simulink model "MCU_SpeedCal"  (R2022b)
settings: Solver=FixedStepDiscrete  StartTime=0.0  StopTime=10.0  RelTol=1e-3
undefined symbols (not defined in the file or in its folder): ParamCfg_RotateNp_u16, ParamCfg_ZeroTorqueNoworkSpeed_u16, ParamCfg_ZeroTorqueWorkSpeed_u16, POWER_ON
libraries: simulink x3
settings Model: DataDictionary=MCU_SpeedCal_Sldd.sldd  Creator=ZYH  LastModifiedBy=ZYH
settings OptimizationCC: DefaultParameterBehavior=Inlined  EnhancedBackFolding=on  PassReuseOutputArgsAs=Individual arguments  ZeroExternalMemoryAtStartup=off  ZeroInternalMemoryAtStartup=off  OptimizeBlockOrder=speed  DifferentSizesBufferReuse=on  OptimizationCustomize=off  EfficientTunableParamExpr=on
settings DebuggingCC: ParameterTunabilityLossMsg=error
settings SFSimCC: MATLABDynamicMemAlloc=off
settings RTWCC: Description=Embedded Coder  SystemTargetFile=ert.tlc  GenCodeOnly=on  TemplateMakefile=ert_default_tmf
settings CodeAppCC: ForceParamTrailComments=on  IgnoreCustomStorageClasses=off  OperatorAnnotations=on  SimulinkDataObjDesc=on  SFDataObjDesc=on  InsertBlockDesc=on
settings ERTTargetCC: TargetLangStandard=C99 (ISO)  GenerateSampleERTMain=on  InlinedParameterPlacement=NonHierarchical  ERTCustomFileTemplate=example_file_process.tlc

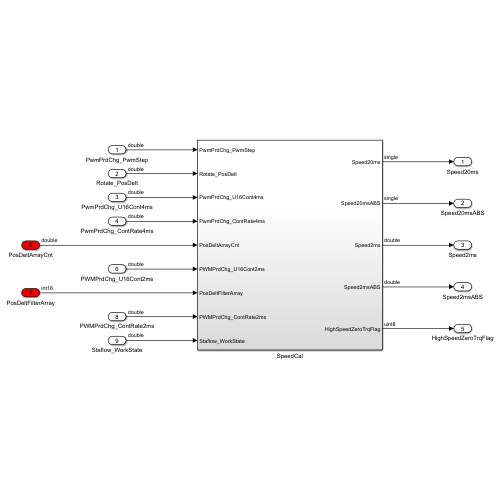
[thumbnail: Simulink's stored preview of the top-level diagram]
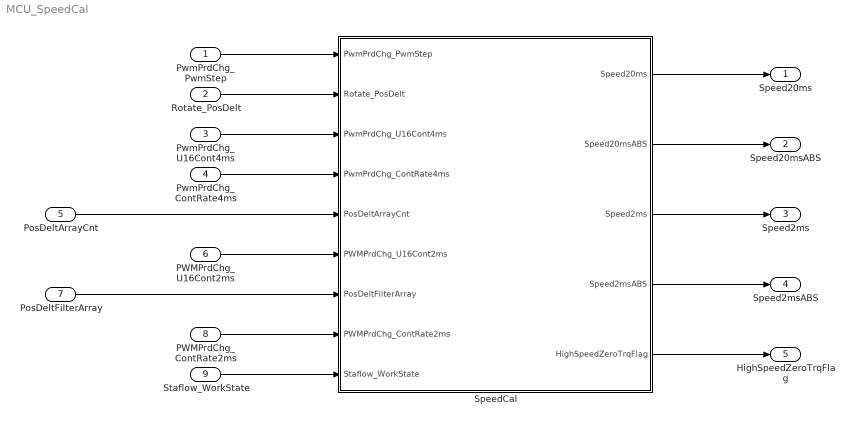
== system MCU_SpeedCal ==
  PwmPrdChg_PwmStep : Inport
  Rotate_PosDelt : Inport  Port=2
  PwmPrdChg_U16Cont4ms : Inport  Port=3
  PwmPrdChg_ContRate4ms : Inport  Port=4
  PosDeltArrayCnt : Inport  Port=5
  PWMPrdChg_U16Cont2ms : Inport  Port=6
  PosDeltFilterArray : Inport  Port=7
  PWMPrdChg_ContRate2ms : Inport  Port=8
  Staflow_WorkState : Inport  Port=9
  SpeedCal : Subsystem
  Speed20ms : Outport
  Speed20msABS : Outport  Port=2
  Speed2ms : Outport  Port=3
  Speed2msABS : Outport  Port=4
  HighSpeedZeroTrqFlag : Outport  Port=5
  wires:
  PwmPrdChg_PwmStep/1 -> SpeedCal/1(PwmPrdChg_PwmStep)
  Rotate_PosDelt/1 -> SpeedCal/2(Rotate_PosDelt)
  PwmPrdChg_U16Cont4ms/1 -> SpeedCal/3(PwmPrdChg_U16Cont4ms)
  PwmPrdChg_ContRate4ms/1 -> SpeedCal/4(PwmPrdChg_ContRate4ms)
  PosDeltArrayCnt/1 -> SpeedCal/5(PosDeltArrayCnt)
  PWMPrdChg_U16Cont2ms/1 -> SpeedCal/6(PWMPrdChg_U16Cont2ms)
  PosDeltFilterArray/1 -> SpeedCal/7(PosDeltFilterArray)
  PWMPrdChg_ContRate2ms/1 -> SpeedCal/8(PWMPrdChg_ContRate2ms)
  SpeedCal/1(Speed20ms) -> Speed20ms/1
  SpeedCal/2(Speed20msABS) -> Speed20msABS/1
  SpeedCal/3(Speed2ms) -> Speed2ms/1
  SpeedCal/4(Speed2msABS) -> Speed2msABS/1
  SpeedCal/5(HighSpeedZeroTrqFlag) -> HighSpeedZeroTrqFlag/1
  Staflow_WorkState/1 -> SpeedCal/9(Staflow_WorkState)

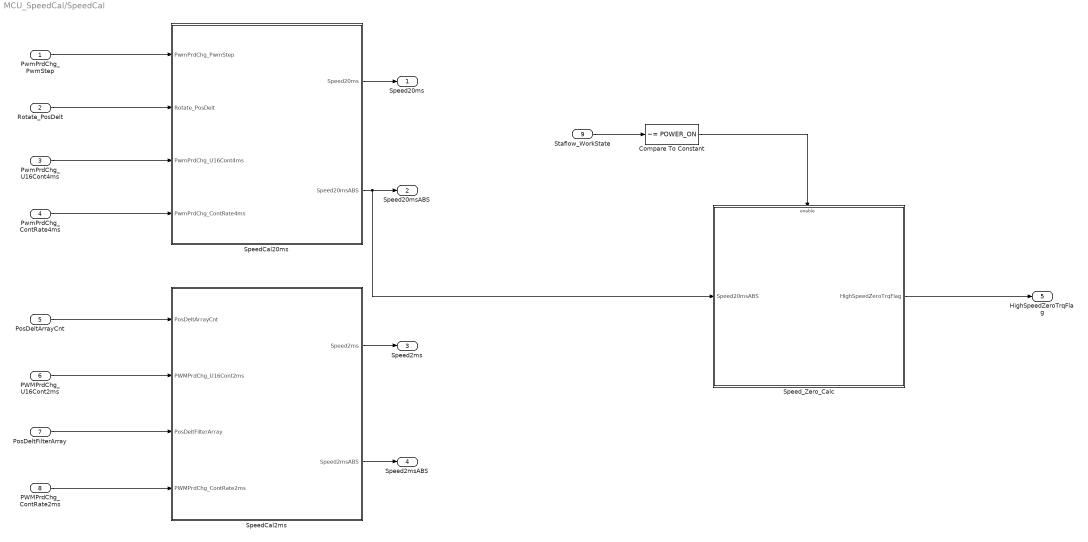
== system MCU_SpeedCal/SpeedCal ==
  PwmPrdChg_PwmStep : Inport
  Rotate_PosDelt : Inport  Port=2
  PwmPrdChg_U16Cont4ms : Inport  Port=3
  PwmPrdChg_ContRate4ms : Inport  Port=4
  PosDeltArrayCnt : Inport  Port=5
  PWMPrdChg_U16Cont2ms : Inport  Port=6
  PosDeltFilterArray : Inport  Port=7
  PWMPrdChg_ContRate2ms : Inport  Port=8
  Staflow_WorkState : Inport  Port=9
  Compare To Constant : simulink/Logic and Bit Operations/Compare To Constant  relop=~=  const=POWER_ON  OutDataTypeStr=boolean
  SpeedCal20ms : Subsystem
  SpeedCal2ms : Subsystem
  Speed_Zero_Calc : Subsystem
  Speed20ms : Outport
  Speed20msABS : Outport  Port=2
  Speed2ms : Outport  Port=3
  Speed2msABS : Outport  Port=4
  HighSpeedZeroTrqFlag : Outport  Port=5
  wires:
  PwmPrdChg_PwmStep/1 -> SpeedCal20ms/1(PwmPrdChg_PwmStep)
  Rotate_PosDelt/1 -> SpeedCal20ms/2(Rotate_PosDelt)
  PwmPrdChg_U16Cont4ms/1 -> SpeedCal20ms/3(PwmPrdChg_U16Cont4ms)
  PwmPrdChg_ContRate4ms/1 -> SpeedCal20ms/4(PwmPrdChg_ContRate4ms)
  SpeedCal20ms/1(Speed20ms) -> Speed20ms/1
  SpeedCal20ms/2(Speed20msABS) -> Speed20msABS/1, Speed_Zero_Calc/1(Speed20msABS)
  PosDeltArrayCnt/1 -> SpeedCal2ms/1(PosDeltArrayCnt)
  PWMPrdChg_U16Cont2ms/1 -> SpeedCal2ms/2(PWMPrdChg_U16Cont2ms)
  PosDeltFilterArray/1 -> SpeedCal2ms/3(PosDeltFilterArray)
  PWMPrdChg_ContRate2ms/1 -> SpeedCal2ms/4(PWMPrdChg_ContRate2ms)
  SpeedCal2ms/2(Speed2msABS) -> Speed2msABS/1
  SpeedCal2ms/1(Speed2ms) -> Speed2ms/1
  Speed_Zero_Calc/1(HighSpeedZeroTrqFlag) -> HighSpeedZeroTrqFlag/1
  Staflow_WorkState/1 -> Compare To Constant/1
  Compare To Constant/1 -> Speed_Zero_Calc/Enable

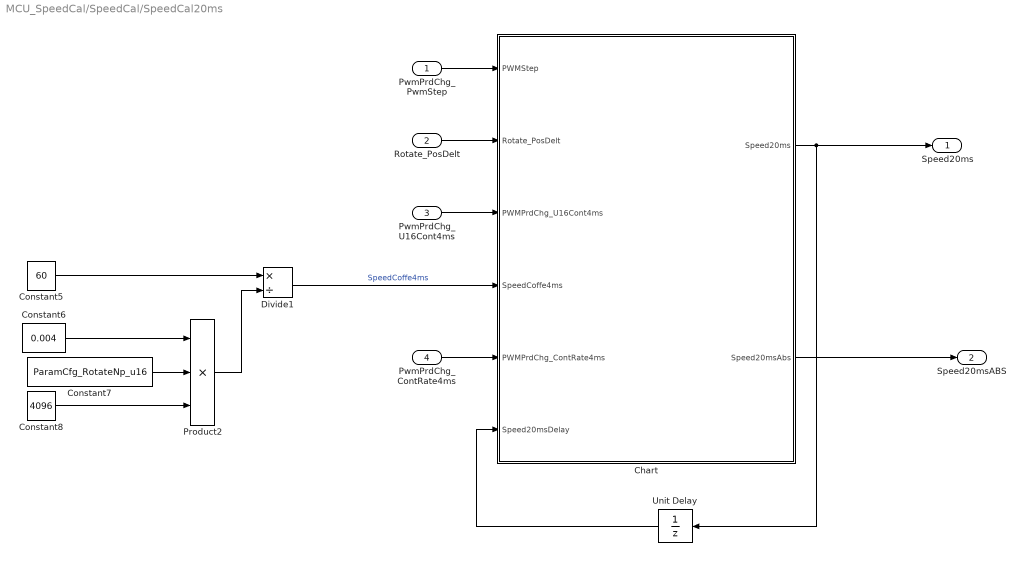
== system MCU_SpeedCal/SpeedCal/SpeedCal20ms ==
  PwmPrdChg_PwmStep : Inport
  Rotate_PosDelt : Inport  Port=2
  PwmPrdChg_U16Cont4ms : Inport  Port=3
  PwmPrdChg_ContRate4ms : Inport  Port=4
  Chart : Stateflow chart  TreatAsAtomicUnit=on
  Constant5 : Constant  Value=60  OutDataTypeStr=single
  Constant6 : Constant  Value=0.004  OutDataTypeStr=single
  Constant7 : Constant  Value=ParamCfg_RotateNp_u16  OutDataTypeStr=uint16
  Constant8 : Constant  Value=4096
  Divide1 : Product  Inputs=*/
  Product2 : Product  Inputs=3
  Unit Delay : UnitDelay  SampleTime=-1  HasFrameUpgradeWarning=on
  Speed20ms : Outport
  Speed20msABS : Outport  Port=2
  wires:
  PwmPrdChg_PwmStep/1 -> Chart/1(PWMStep)
  Rotate_PosDelt/1 -> Chart/2(Rotate_PosDelt)
  PwmPrdChg_U16Cont4ms/1 -> Chart/3(PWMPrdChg_U16Cont4ms)
  Chart/2(Speed20msAbs) -> Speed20msABS/1
  PwmPrdChg_ContRate4ms/1 -> Chart/5(PWMPrdChg_ContRate4ms)
  Constant5/1 -> Divide1/1
  Constant6/1 -> Product2/1
  Constant7/1 -> Product2/2
  Product2/1 -> Divide1/2
  Constant8/1 -> Product2/3
  Divide1/1 -> Chart/4(SpeedCoffe4ms)  "SpeedCoffe4ms"
  Chart/1(Speed20ms) -> Speed20ms/1, Unit Delay/1
  Unit Delay/1 -> Chart/6(Speed20msDelay)

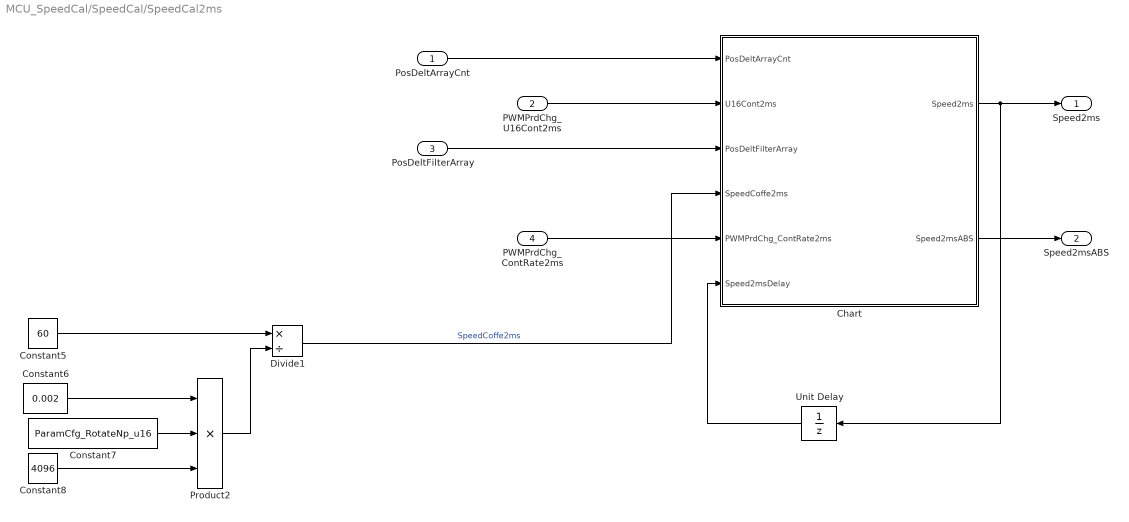
== system MCU_SpeedCal/SpeedCal/SpeedCal2ms ==
  PosDeltArrayCnt : Inport
  PWMPrdChg_U16Cont2ms : Inport  Port=2
  PosDeltFilterArray : Inport  Port=3
  PWMPrdChg_ContRate2ms : Inport  Port=4
  Chart : Stateflow chart  TreatAsAtomicUnit=on
  Constant5 : Constant  Value=60  OutDataTypeStr=single
  Constant6 : Constant  Value=0.002  OutDataTypeStr=single
  Constant7 : Constant  Value=ParamCfg_RotateNp_u16  OutDataTypeStr=uint16
  Constant8 : Constant  Value=4096
  Divide1 : Product  Inputs=*/
  Product2 : Product  Inputs=3
  Unit Delay : UnitDelay  SampleTime=-1  HasFrameUpgradeWarning=on
  Speed2ms : Outport
  Speed2msABS : Outport  Port=2
  wires:
  PosDeltArrayCnt/1 -> Chart/1(PosDeltArrayCnt)
  PWMPrdChg_U16Cont2ms/1 -> Chart/2(U16Cont2ms)
  Product2/1 -> Divide1/2
  Constant7/1 -> Product2/2
  Constant8/1 -> Product2/3
  Constant6/1 -> Product2/1
  Divide1/1 -> Chart/4(SpeedCoffe2ms)  "SpeedCoffe2ms"
  Constant5/1 -> Divide1/1
  PosDeltFilterArray/1 -> Chart/3(PosDeltFilterArray)
  PWMPrdChg_ContRate2ms/1 -> Chart/5(PWMPrdChg_ContRate2ms)
  Chart/1(Speed2ms) -> Unit Delay/1, Speed2ms/1
  Unit Delay/1 -> Chart/6(Speed2msDelay)
  Chart/2(Speed2msABS) -> Speed2msABS/1

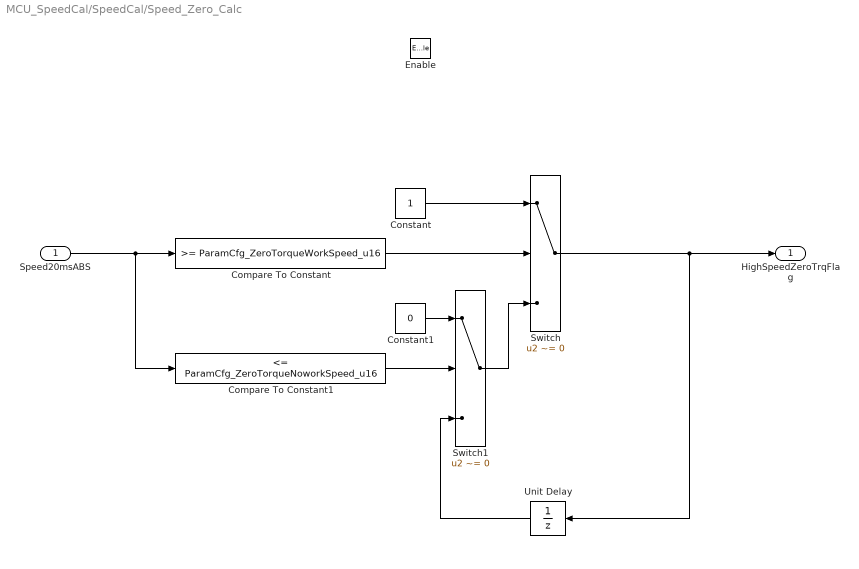
== system MCU_SpeedCal/SpeedCal/Speed_Zero_Calc ==
  Speed20msABS : Inport
  Enable : EnablePort
  Compare To Constant : simulink/Logic and Bit Operations/Compare To Constant  relop=>=  const=ParamCfg_ZeroTorqueWorkSpeed_u16  OutDataTypeStr=boolean
  Compare To Constant1 : simulink/Logic and Bit Operations/Compare To Constant  relop=<=  const=ParamCfg_ZeroTorqueNoworkSpeed_u16  OutDataTypeStr=boolean
  Constant : Constant  OutDataTypeStr=uint8
  Constant1 : Constant  Value=0  OutDataTypeStr=uint8
  Switch : Switch  Criteria=u2 ~= 0  SaturateOnIntegerOverflow=off  InputSameDT=off
  Switch1 : Switch  Criteria=u2 ~= 0  SaturateOnIntegerOverflow=off  InputSameDT=off
  Unit Delay : UnitDelay  SampleTime=-1  HasFrameUpgradeWarning=on
  HighSpeedZeroTrqFlag : Outport
  wires:
  Speed20msABS/1 -> Compare To Constant1/1, Compare To Constant/1
  Compare To Constant/1 -> Switch/2
  Switch/1 -> Unit Delay/1, HighSpeedZeroTrqFlag/1
  Constant/1 -> Switch/1
  Switch1/1 -> Switch/3
  Compare To Constant1/1 -> Switch1/2
  Constant1/1 -> Switch1/1
  Unit Delay/1 -> Switch1/3

== stateflow chart MCU_SpeedCal/SpeedCal/SpeedCal2ms/Chart ==
  (default) -> (junction 2) : {ArrayCnt = PosDeltArrayCnt}
  (junction 2) -> (junction 4) [order 1] : [ArrayCnt == 0]{ArrayCnt = 39}
  (junction 2) -> (junction 4) [order 2] : {ArrayCnt = ArrayCnt -1}
  (junction 4) -> (junction 33)
  (junction 33) -> (junction 35) : {index=0;}
  (junction 35) -> (junction 34) [order 1] : [index<U16Cont2ms]
  (junction 34) -> (junction 56)
  (junction 37) -> (junction 35)
  (junction 35) -> (junction 38) [order 2] : {
      | SpeedNew = Rotate_Delt_Add_2ms*SpeedCoffe2ms*PWMPrdChg_ContRate2ms;
      | Rotate_Delt_Add_2ms = 0;
      |
      |
      | SpeedOld = Speed2msDelay
      | Speed2ms = SpeedOld*0.9 + SpeedNew*0.1;
      | Speed2msABS = abs(Speed2ms);
      | }
  (junction 56) -> (junction 57) [order 1] : [index<=ArrayCnt]
  (junction 56) -> (junction 58) [order 2] : {j = ArrayCnt+40-i;}
  (junction 57) -> (junction 59) : {j = ArrayCnt-index;}
  (junction 59) -> (junction 58)
  (junction 58) -> (junction 36) : {
      | Rotate_Delt_Add_2ms =PosDeltFilterArray[j]
      | }
  (junction 36) -> (junction 37) : {index=index+1;}
  data: PosDeltArrayCnt input; U16Cont2ms input; i local double; j local double; Rotate_Delt_Add_2ms local double; index local double; PosDeltFilterArray input int16 size=40; ArrayCnt local uint16 =0; SpeedOld local single =0; SpeedNew local single =0; SpeedCoffe2ms input; PWMPrdChg_ContRate2ms input; Speed2msDelay input; Speed2ms output double; Speed2msABS output double

== stateflow chart MCU_SpeedCal/SpeedCal/SpeedCal20ms/Chart ==
  (default) -> (junction 1)
  (junction 1) -> (junction 4) [order 2]
  (junction 1) -> (junction 4) [order 1] : [PWMStep == 4]
      | {Cont4ms=0;RotateDeltAdd4ms=0}
  (junction 4) -> (junction 9) : {
      | Cont4ms = Cont4ms+1;
      | RotateDeltAdd4ms = RotateDeltAdd4ms+Rotate_PosDelt
      | }
  (junction 9) -> (junction 12) [order 1] : [Cont4ms>PWMPrdChg_U16Cont4ms]
  (junction 9) -> (junction 30) [order 2]
  (junction 12) -> (junction 15) : {
      | SpeedNew = (RotateDeltAdd4ms*SpeedCoffe4ms)*PWMPrdChg_ContRate4ms;
      | Cont4ms = 0;
      | RotateDeltAdd4ms = 0;
      | SpeedOld = Speed20ms;
      | Speed20ms = SpeedOld*0.9 + SpeedNew*0.1
      | }
  (junction 15) -> (junction 21) [order 1] : [abs(Speed20ms)<0.1]{Speed20ms = 0}
  (junction 15) -> (junction 21) [order 2]
  (junction 21) -> (junction 27) : {Speed20msAbs = abs(Speed20ms)}
  (junction 27) -> (junction 30)
  (junction 30) -> (junction 33)
  data: PWMStep input; Cont4ms local uint16 size=1 =0; RotateDeltAdd4ms local int64 size=1 =0; Rotate_PosDelt input; PWMPrdChg_U16Cont4ms input; SpeedNew local single size=1 =0; SpeedCoffe4ms input; PWMPrdChg_ContRate4ms input; SpeedOld local single size=1 =0; Speed20ms output single =0; Speed20msDelay input; Speed20msAbs output single
